simulink subsystem "massBalanceUnit"  (R2024a)
settings: Solver=VariableStepAuto  StartTime=0.0  StopTime=10.0  RelTol=1e-3
settings Model: Creator=ilan.malkin  LastModifiedBy=jason.miskin

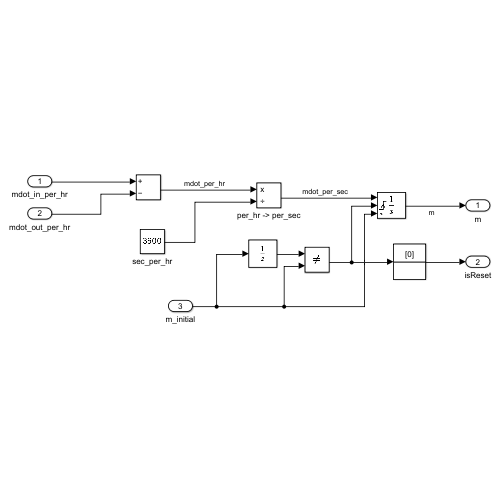
[thumbnail: Simulink's stored preview of the top-level diagram]
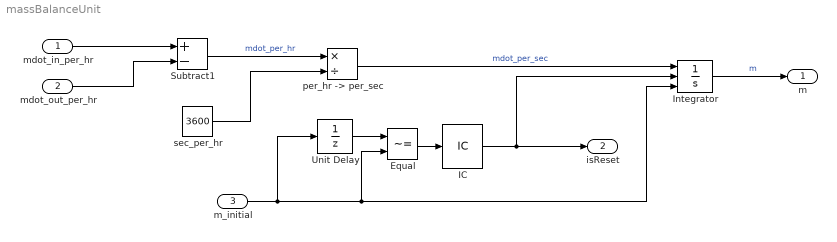
== system massBalanceUnit ==
  mdot_in_per_hr : Inport
  mdot_out_per_hr : Inport  Port=2
  m_initial : Inport  Port=3
  Equal : RelationalOperator  Operator=~=  OutDataTypeStr=boolean  RndMeth=Simplest  InputSameDT=off
  IC : InitialCondition  Value=0
  Integrator : Integrator  ExternalReset=rising  InitialConditionSource=external
  Subtract1 : Sum  Inputs=+-
  Unit Delay : UnitDelay  SampleTime=-1  HasFrameUpgradeWarning=on
  "per_hr -> per_sec" : Product  Inputs=*/
  sec_per_hr : Constant  Value=3600
  m : Outport
  isReset : Outport  Port=2
  wires:
  Integrator/1 -> m/1  "m"
  Subtract1/1 -> "per_hr -> per_sec"/1  "mdot_per_hr"
  mdot_out_per_hr/1 -> Subtract1/2
  m_initial/1 -> Unit Delay/1, Integrator/3, Equal/2
  mdot_in_per_hr/1 -> Subtract1/1
  sec_per_hr/1 -> "per_hr -> per_sec"/2
  "per_hr -> per_sec"/1 -> Integrator/1  "mdot_per_sec"
  Unit Delay/1 -> Equal/1
  Equal/1 -> IC/1
  IC/1 -> Integrator/2, isReset/1
